simulink model "First_order"  (R2021a)
settings: Solver=FixedStepDiscrete  StartTime=0.0  StopTime=inf  FixedStep=1e-3  MaxStep=1e-3  RelTol=1e-3  EnableMultiTasking=on
libraries: arduinolib x4
settings Model: SILPILModeSetting=veronly  ExtModeTrigDuration=2  Creator=Beshary  LastModifiedBy=Beshary
settings DataIOCC: InspectSignalLogs=on
settings OptimizationCC: EnhancedBackFolding=on  PassReuseOutputArgsAs=Individual arguments  ZeroExternalMemoryAtStartup=off  ZeroInternalMemoryAtStartup=off  MaxStackSize=64  OptimizeBlockOrder=speed  DifferentSizesBufferReuse=on  OptimizationCustomize=off  EfficientTunableParamExpr=on
settings DebuggingCC: ParameterTunabilityLossMsg=error
settings HardwareCC: ProdBitPerInt=16  ProdBitPerPointer=16  ProdBitPerSizeT=16  ProdBitPerPtrDiffT=16  ProdLargestAtomicFloat=None  ProdWordSize=8  ProdHWDeviceType=Atmel->AVR
settings SFSimCC: MATLABDynamicMemAlloc=off
settings RTWCC: SystemTargetFile=ert.tlc  HardwareBoard=Arduino Uno  TemplateMakefile=ert_default_tmf  Toolchain=Arduino AVR  BuildConfiguration=Faster Runs
settings CodeAppCC: ForceParamTrailComments=on  IgnoreCustomStorageClasses=off  OperatorAnnotations=on  SimulinkDataObjDesc=on  SFDataObjDesc=on  InsertBlockDesc=on
settings ERTTargetCC: SupportContinuousTime=on  SupportVariableSizeSignals=on  ExtModeStaticAllocSize=250

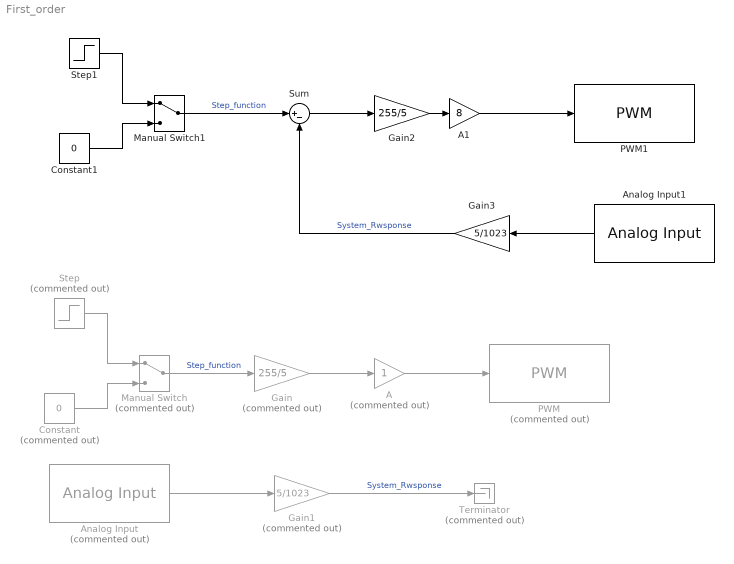
== system First_order ==
  A : Gain  Commented=on
  A1 : Gain  Gain=8
  Analog Input : arduinolib/Analog Input  Commented=on  pinNumber=0  ReadResultsOnly=off  ConversionTriggerSource=Software  ExternalTriggerType=uint32( 0 )  OutputDataType=uint16  EnableConversionCompleteNotify=off  EnableOuputStatus=off  SampleTime=-1  blockPlatform=arduino
  Analog Input1 : arduinolib/Analog Input  pinNumber=0  ReadResultsOnly=off  ConversionTriggerSource=Software  ExternalTriggerType=uint32( 0 )  OutputDataType=uint16  EnableConversionCompleteNotify=off  EnableOuputStatus=off  SampleTime=-1  blockPlatform=arduino
  Constant : Constant  Commented=on  Value=0
  Constant1 : Constant  Value=0
  Gain : Gain  Commented=on  Gain=255/5
  Gain1 : Gain  Commented=on  Gain=5/1023
  Gain2 : Gain  Gain=255/5
  Gain3 : Gain  Gain=5/1023
  Manual Switch : ManualSwitch  Commented=on
  Manual Switch1 : ManualSwitch
  PWM : arduinolib/PWM  Commented=on  pinNumber=9  frequencyType=Default  desiredFrequency=490.2  achievableFrequency=490.2
  PWM1 : arduinolib/PWM  pinNumber=9  frequencyType=Default  desiredFrequency=490.2  achievableFrequency=490.2
  Step : Step  Commented=on  After=5  SampleTime=0
  Step1 : Step  After=4  SampleTime=0
  Sum : Sum  Inputs=|+-
  Terminator : Terminator  Commented=on
  wires:
  Manual Switch/1 -> Gain/1  "Step_function"
  Step/1 -> Manual Switch/1
  Constant/1 -> Manual Switch/2
  Analog Input/1 -> Gain1/1
  Gain1/1 -> Terminator/1  "System_Rwsponse"
  Gain/1 -> A/1
  A/1 -> PWM/1
  A1/1 -> PWM1/1
  Gain2/1 -> A1/1
  Gain3/1 -> Sum/2  "System_Rwsponse"
  Constant1/1 -> Manual Switch1/2
  Step1/1 -> Manual Switch1/1
  Manual Switch1/1 -> Sum/1  "Step_function"
  Analog Input1/1 -> Gain3/1
  Sum/1 -> Gain2/1
